simulink model "modelo_ss"  (R2020a)
settings: Solver=FixedStepAuto  StartTime=0.0  StopTime=2  FixedStep=1e-3  RelTol=1e-3
settings Model: Creator=xiz12  LastModifiedBy=gusta
settings DebuggingCC: UnconnectedInputMsg=none  UnconnectedOutputMsg=none  UnconnectedLineMsg=none  SFMachineParentedDataDiag=error

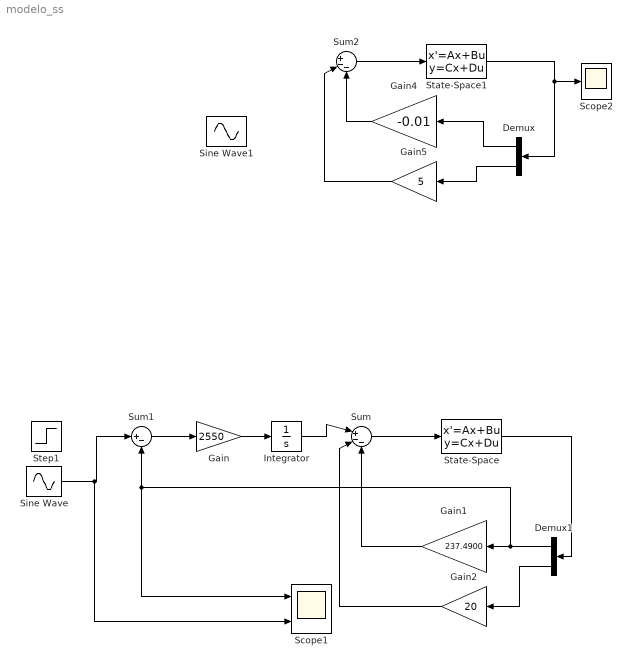
== system modelo_ss ==
  Demux : Demux  Outputs=2
  Demux1 : Demux  Outputs=2
  Gain : Gain  Gain=2550
  Gain1 : Gain  Gain=237.4900
  Gain2 : Gain  Gain=20
  Gain4 : Gain  Gain=-0.01
  Gain5 : Gain  Gain=5
  Integrator : Integrator
  Scope1 : Scope  NumInputPorts=2
  Scope2 : Scope
  Sine Wave : Sin  Amplitude=80  Frequency=10  SampleTime=0
  Sine Wave1 : Sin  SampleTime=0
  State-Space : StateSpace  A=[-10 1;-0.02 -2]  B=[0;2]  C=[1 0;0 1]  D=[0;0]  InitialCondition=[0 0]
  State-Space1 : StateSpace  A=[-10 1;-0.02 -2]  B=[0;2]  C=[1 0;0 1]  D=[0;0]  InitialCondition=[1000 0]
  Step1 : Step  Time=0.4  After=105  SampleTime=0
  Sum : Sum  Inputs=|+--
  Sum1 : Sum  Inputs=|+-
  Sum2 : Sum  Inputs=|+--
  wires:
  Gain1/1 -> Sum/3
  Gain2/1 -> Sum/2
  Sum/1 -> State-Space/1
  Gain/1 -> Integrator/1
  Sum1/1 -> Gain/1
  Integrator/1 -> Sum/1
  Gain4/1 -> Sum2/3
  Gain5/1 -> Sum2/2
  Sum2/1 -> State-Space1/1
  State-Space1/1 -> Scope2/1, Demux/1
  Demux/1 -> Gain4/1
  Demux/2 -> Gain5/1
  Demux1/1 -> Scope1/1, Sum1/2, Gain1/1
  Demux1/2 -> Gain2/1
  State-Space/1 -> Demux1/1
  Sine Wave/1 -> Scope1/2, Sum1/1
